simulink model "REL"  (R2022a)
settings: Solver=FixedStepDiscrete  StartTime=0.0  StopTime=10.0  FixedStep=0.01  RelTol=1e-3
libraries: simulink x4, DoorRatSts x4, DoorRlsDriver x4, DoorRlsReq x4
(part 2 of 2)

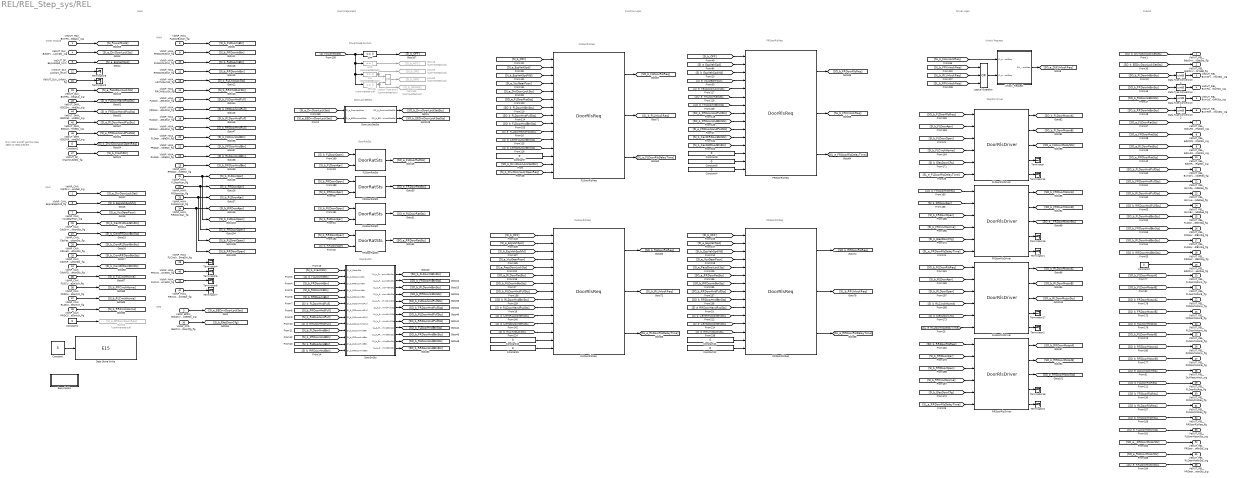
== system REL/REL_Step_sys/REL ==
  note: Only NFC and BT got this Req
      | //830 no need present
  note: CAN
  note: HWA
  note: Function Logic
  note: Input
  note: Output
  note: Input Preprocess
  note: Other Module
  note: CFG
  note: PowerMode Divition
  note: DoorLockSetSts
  note: DoorRatSts
  note: Driver Logic
  note: Unlock Request
  note: DoorRls Driver
  note: FLDoorRlsReq
  note: FRDoorRlsReq
  note: RLDoorRlsReq
  note: RRDoorRlsReq
  note: DoorSwSts
  VeOUT_PDU_BcmPowerStatusFeedback_sig : Inport
  VeINP_CAN_CdcDrvrDoorLockSet_sig : Inport  Port=2
  VeINP_EPRM_BdcDrvrDoorLockSetSts_sig : Inport  Port=3
  VeOUT_DLK_BdcDrvrDoorLockSts_sig : Inport  Port=4
  VeOUT_SP_EspVehSpd_kmh : Inport  Port=5
  VbINP_CAN_EspVehSpdVld_flg : Inport  Port=6
  VeINP_CAN_VcuGearPosn_sig : Inport  Port=7
  VbINP_HWA_FLDoorButton_flg : Inport  Port=8
  VbINP_HWA_FRDoorButton_flg : Inport  Port=9
  VbINP_HWA_RLDoorButton_flg : Inport  Port=10
  VbINP_HWA_RRDoorButton_flg : Inport  Port=11
  VmOUT_DLK_LockSrc_enum : Inport  Port=12
  VbINP_HWA_LRChildLckSt_flg : Inport  Port=13
  VbINP_HWA_RRChildLckSt_flg : Inport  Port=14
  VbOUT_DLK_Unlock_flg : Inport  Port=15
  VbINP_HWA_FLDoorOutButton_flg : Inport  Port=16
  VbINP_HWA_FRDoorOutButton_flg : Inport  Port=17
  VbINP_HWA_RLDoorOutButton_flg : Inport  Port=18
  VbINP_HWA_RRDoorOutButton_flg : Inport  Port=19
  VbINP_HWA_FLDoorHandleSW_flg : Inport  Port=20
  VbINP_HWA_FRDoorHandleSW_flg : Inport  Port=21
  VbINP_HWA_RLDoorHandleSW_flg : Inport  Port=22
  VbINP_HWA_RRDoorHandleSW_flg : Inport  Port=23
  VbINP_CAN_CdcAllDoorOpenButtonSts_flg : Inport  Port=24
  VeOUT_DLK_BCMPassengerDoorLockStatus_sig : Inport  Port=25
  VbINP_CAN_CdcDrvrDoorButtonSts_flg : Inport  Port=26
  VbINP_CAN_CdcPassDoorButtonSts_flg : Inport  Port=27
  VbINP_CAN_CdcLeReDoorButtonSts_flg : Inport  Port=28
  VbINP_CAN_CdcRiReDoorButtonSts_flg : Inport  Port=29
  VbINP_CFG_ElectricalDoorCfg_flg : Inport  Port=30
  VbINP_HWA_FLDoorAjar_flg : Inport  Port=31
  VbINP_HWA_FRDoorAjar_flg : Inport  Port=32
  VbINP_HWA_RLDoorAjar_flg : Inport  Port=33
  VbINP_HWA_RRDoorAjar_flg : Inport  Port=34
  VbINP_CAN_FLDCUCinchHomeSwitch_flg : Inport  Port=35
  VbINP_CAN_FRDCUCinchHomeSwitch_flg : Inport  Port=36
  VbINP_CAN_RLDCUCinchHomeSwitch_flg : Inport  Port=37
  VbINP_CAN_RRDCUCinchHomeSwitch_flg : Inport  Port=38
  VbINP_HWA_FLCinchHomeSW_flg : Inport  Port=39
  VbINP_HWA_FRCinchHomeSW_flg : Inport  Port=40
  VbINP_HWA_RLCinchHomeSW_flg : Inport  Port=41
  VbINP_HWA_RRCinchHomeSW_flg : Inport  Port=42
  VeOUT_DHM_BDCDrvrDoorHndSts_sig : Inport  Port=43
  VeOUT_DHM_BDCPassDoorHndSts_sig : Inport  Port=44
  VeOUT_DHM_BDCLeReDoorHndSts_sig : Inport  Port=45
  VeOUT_DHM_BDCRiReDoorHndSts_sig : Inport  Port=46
  VbOUT_SP_CrashOutpSts_flg : Inport  Port=47
  ACC : simulink/Logic and Bit Operations/Compare To Constant  Commented=on  relop===  const=1  OutDataTypeStr=boolean
  Constant : Constant  Value=5
  Constant1 : Constant  Value=0  OutDataTypeStr=uint8
  Constant{2..4,6..12} (10 alike) : Constant  Value=0  OutDataTypeStr=boolean
  Data Store Write : DataStoreWrite  DataStoreName=E15  IndexOptions=Index vector (dialog)  Indices=1  OutputSizes=1
  Data Type Conversion{,1..2,4} (4 alike) : DataTypeConversion  OutDataTypeStr=uint8  SaturateOnIntegerOverflow=off  RndMeth=Floor
  DoorLockSetSts : Stateflow chart  TreatAsAtomicUnit=on
  DoorSwSts : Stateflow chart  TreatAsAtomicUnit=on
  FLDoorRatSts : DoorRatSts/DoorRatSts  SystemSampleTime=-1  VariantActivationTime=update diagram  Latency=0  AutoFrameSizeCalculation=off
  FLDoorRlsDriver : DoorRlsDriver/DoorRlsDriver  SystemSampleTime=-1  VariantActivationTime=update diagram  Latency=0  AutoFrameSizeCalculation=off
  FLDoorRlsReq : DoorRlsReq/DoorRlsReq  SystemSampleTime=-1  VariantActivationTime=update diagram  Latency=0  AutoFrameSizeCalculation=off
  FRDoorRatSts : DoorRatSts/DoorRatSts  SystemSampleTime=-1  VariantActivationTime=update diagram  Latency=0  AutoFrameSizeCalculation=off
  FRDoorRlsDriver : DoorRlsDriver/DoorRlsDriver  SystemSampleTime=-1  VariantActivationTime=update diagram  Latency=0  AutoFrameSizeCalculation=off
  FRDoorRlsReq : DoorRlsReq/DoorRlsReq  SystemSampleTime=-1  VariantActivationTime=update diagram  Latency=0  AutoFrameSizeCalculation=off
  GRANK : simulink/Logic and Bit Operations/Compare To Constant  Commented=on  relop===  const=3  OutDataTypeStr=boolean
  Goto106 : Goto  Commented=on  GotoTag=SI_b_GRANK
  Goto48 : Goto  Commented=on  GotoTag=SI_b_ACC
  Goto56 : Goto  Commented=on  GotoTag=SI_e_BTDoorOpenReq
  Goto58 : Goto  Commented=on  GotoTag=SI_b_ON
  Goto69 : Goto  Commented=on  GotoTag=SI_b_IGN
  Logical Operator3 : Logic  Commented=on  Operator=OR  AllPortsSameDT=off  OutDataTypeStr=boolean
  Logical Operator : Logic  Operator=OR  Inputs=3  OutDataTypeStr=boolean
  "OFF " : simulink/Logic and Bit Operations/Compare To Constant  relop===  const=0  OutDataTypeStr=boolean
  ON : simulink/Logic and Bit Operations/Compare To Constant  Commented=on  relop===  const=2  OutDataTypeStr=boolean
  RLDoorRatSts : DoorRatSts/DoorRatSts  SystemSampleTime=-1  VariantActivationTime=update diagram  Latency=0  AutoFrameSizeCalculation=off
  RLDoorRlsDriver : DoorRlsDriver/DoorRlsDriver  SystemSampleTime=-1  VariantActivationTime=update diagram  Latency=0  AutoFrameSizeCalculation=off
  RLDoorRlsReq : DoorRlsReq/DoorRlsReq  SystemSampleTime=-1  VariantActivationTime=update diagram  Latency=0  AutoFrameSizeCalculation=off
  RRDoorRatSts : DoorRatSts/DoorRatSts  SystemSampleTime=-1  VariantActivationTime=update diagram  Latency=0  AutoFrameSizeCalculation=off
  RRDoorRlsDriver : DoorRlsDriver/DoorRlsDriver  SystemSampleTime=-1  VariantActivationTime=update diagram  Latency=0  AutoFrameSizeCalculation=off
  RRDoorRlsReq : DoorRlsReq/DoorRlsReq  SystemSampleTime=-1  VariantActivationTime=update diagram  Latency=0  AutoFrameSizeCalculation=off
  Recycle Bin : Subsystem
  Terminator{,1..9,15..18} (14 alike) : Terminator
  Unlock_Request : Stateflow chart  TreatAsAtomicUnit=on
  VbOUT_REL_BdcDrvrDoorLockSetSts_flg : Outport
  VbOUT_REL_BdcDrvrDoorLockSetStsToEE_flg : Outport  Port=2
  VeOUT_REL_BcmDrvrDoorSwtSts_sig : Outport  Port=3
  VeOUT_REL_BcmPassDoorSwtSts_sig : Outport  Port=4  OutDataTypeStr=uint8
  VeOUT_REL_BcmLeReDoorSwtSts_sig : Outport  Port=5  OutDataTypeStr=uint8
  VeOUT_REL_BcmRiReDoorSwtSts_sig : Outport  Port=6  OutDataTypeStr=uint8
  VeOUT_REL_BdcLFDoorRatSts_sig : Outport  Port=7
  VeOUT_REL_BdcRFDoorRatSts_sig : Outport  Port=8
  VeOUT_REL_BdcLRDoorRatSts_sig : Outport  Port=9
  VeOUT_REL_BdcRRDoorRatSts_sig : Outport  Port=10
  VbOUT_REL_BcmDrvrDoorHandleReq_flg : Outport  Port=11
  VbOUT_REL_BcmPassDoorHandleReq_flg : Outport  Port=12
  VbOUT_REL_BcmLeReDoorHandleReq_flg : Outport  Port=13
  VbOUT_REL_BcmBcmRiReDoorHandleReq_flg : Outport  Port=14
  VbOUT_REL_FLDoorHndlBtnSig_flg : Outport  Port=15
  VbOUT_REL_FRDoorHndlBtnSig_flg : Outport  Port=16
  VbOUT_REL_RLDoorHndlBtnSig_flg : Outport  Port=17
  VbOUT_REL_RRDoorHndlBtnSig_flg : Outport  Port=18
  VbOUT_REL_BdcDrvrDoorLockOpenReq_flg : Outport  Port=19
  VbOUT_REL_FLDoorMotorA_flg : Outport  Port=20
  VbOUT_REL_FLDoorMotorB_flg : Outport  Port=21
  VbOUT_REL_FRDoorMotorA_flg : Outport  Port=22
  VbOUT_REL_FRDoorMotorB_flg : Outport  Port=23
  VbOUT_REL_RLDoorMotorA_flg : Outport  Port=24
  VbOUT_REL_RLDoorMotorB_flg : Outport  Port=25
  VbOUT_REL_RRDoorMotorA_flg : Outport  Port=26
  VbOUT_REL_RRDoorMotorB_flg : Outport  Port=27
  VeOUT_REL_DLKReqUnlock_sig : Outport  Port=28
  VbOUT_REL_FLDoorRlsReq_flg : Outport  Port=29
  VbOUT_REL_FRDoorRlsReq_flg : Outport  Port=30
  VbOUT_REL_RLDoorRlsReq_flg : Outport  Port=31
  VbOUT_REL_RRDoorRlsReq_flg : Outport  Port=32
  VeOUT_REL_FLDoorMotorSts_sig : Outport  Port=33
  VeOUT_REL_FRDoorMotorSts_sig : Outport  Port=34
  VeOUT_REL_RLDoorMotorSts_sig : Outport  Port=35
  VeOUT_REL_RRDoorMotorSts_sig : Outport  Port=36
  wires:
  "OFF "/1 -> [SI_b_OFF]
  [SI_PowerMode] -> "OFF "/1, GRANK/1, ON/1, ACC/1
  ON/1 -> Goto58/1, Logical Operator3/1
  GRANK/1 -> Goto106/1, Logical Operator3/2
  Logical Operator3/1 -> Goto69/1
  ACC/1 -> Goto48/1
  VeINP_EPRM_BdcDrvrDoorLockSetSts_sig/1 -> [SI_e_EEDrvrDoorLockSet]
  [SO_b_DrvrDoorLockSetSts] -> VbOUT_REL_BdcDrvrDoorLockSetSts_flg/1
  DoorLockSetSts/1(SO_b_DoorLockSetSts) -> [SO_b_DrvrDoorLockSetSts]
  VeINP_CAN_CdcDrvrDoorLockSet_sig/1 -> [SI_e_DrvDoorLockSet]
  [SI_e_EEDrvrDoorLockSet] -> DoorLockSetSts/2(SI_e_EEDoorLockSet)
  VeOUT_DLK_BdcDrvrDoorLockSts_sig/1 -> [SI_e_DrvDoorLockSts]
  VeOUT_SP_EspVehSpd_kmh/1 -> [SI_e_EspVehSpd]
  VbINP_CAN_EspVehSpdVld_flg/1 -> [SI_b_EspVehSpdVld]
  VbINP_HWA_FLDoorButton_flg/1 -> [SI_b_FLDoorInBtn]
  VeINP_CAN_VcuGearPosn_sig/1 -> [SI_e_VcuGearPosn]
  VeOUT_DLK_BCMPassengerDoorLockStatus_sig/1 -> [SI_e_PassDoorLockSts]
  VbINP_HWA_FRDoorButton_flg/1 -> [SI_b_FRDoorInBtn]
  VbINP_HWA_LRChildLckSt_flg/1 -> [SI_b_RLChildLckSts]
  VbINP_HWA_RRChildLckSt_flg/1 -> [SI_b_RRChildLckSts]
  VbINP_CAN_CdcDrvrDoorButtonSts_flg/1 -> [SI_b_CentFLDoorBtnSts]
  VbINP_CAN_CdcPassDoorButtonSts_flg/1 -> [SI_b_CentFRDoorBtnSts]
  VbINP_CAN_CdcLeReDoorButtonSts_flg/1 -> [SI_b_CentRLDoorBtnSts]
  VbINP_CAN_CdcRiReDoorButtonSts_flg/1 -> [SI_b_CentRRDoorBtnSts]
  VbINP_HWA_RLDoorButton_flg/1 -> [SI_b_RLDoorInBtn]
  VbINP_HWA_RRDoorButton_flg/1 -> [SI_b_RRDoorInBtn]
  VbINP_HWA_FLDoorAjar_flg/1 -> [SI_b_FLDoorOpen], [SI_b_FLDoorAjar]
  VbINP_HWA_FRDoorAjar_flg/1 -> [SI_b_FRDoorOpen], [SI_b_FRDoorAjar]
  VbINP_HWA_RLDoorAjar_flg/1 -> [SI_b_RLDoorOpen], [SI_b_RLDoorAjar]
  VbINP_HWA_RRDoorAjar_flg/1 -> [SI_b_RRDoorOpen], [SI_b_RRDoorAjar]
  [SI_b_FLDoorOpen] -> FLDoorRatSts/1
  [SI_b_RRDoorAjar] -> RRDoorRatSts/2
  [SI_b_RLDoorAjar] -> RLDoorRatSts/2
  [SI_b_FRDoorAjar] -> FRDoorRatSts/2
  [SI_b_FLDoorAjar] -> FLDoorRatSts/2
  [SI_b_FRDoorOpen] -> FRDoorRatSts/1
  [SI_b_RLDoorOpen] -> RLDoorRatSts/1
  [SI_b_RRDoorOpen] -> RRDoorRatSts/1
  [SO_e_FLDoorRatSts] -> VeOUT_REL_BdcLFDoorRatSts_sig/1
  [SO_e_FRDoorRatSts] -> VeOUT_REL_BdcRFDoorRatSts_sig/1
  [SO_e_RLDoorRatSts] -> VeOUT_REL_BdcLRDoorRatSts_sig/1
  [SO_e_RRDoorRatSts] -> VeOUT_REL_BdcRRDoorRatSts_sig/1
  FLDoorRatSts/1 -> [SO_e_FLDoorRatSts]
  FRDoorRatSts/1 -> [SO_e_FRDoorRatSts]
  RRDoorRatSts/1 -> [SO_e_RRDoorRatSts]
  RLDoorRatSts/1 -> [SO_e_RLDoorRatSts]
  [SO_b_FRDoorInBtnSts] -> Data Type Conversion/1
  [SO_b_RLDoorInBtnSts] -> Data Type Conversion1/1
  [SO_b_RRDoorInBtnSts] -> Data Type Conversion2/1
  [SO_e_DLKUnlockReq] -> VeOUT_REL_DLKReqUnlock_sig/1
  VbINP_HWA_FLDoorHandleSW_flg/1 -> [SI_b_FLDoorHndBtn]
  VbINP_HWA_FRDoorHandleSW_flg/1 -> [SI_b_FRDoorHndBtn]
  VbINP_HWA_RLDoorHandleSW_flg/1 -> [SI_b_RLDoorHndBtn]
  VbINP_HWA_RRDoorHandleSW_flg/1 -> [SI_b_RRDoorHndBtn]
  [SO_b_FLDoorHndPullSts] -> VbOUT_REL_BcmDrvrDoorHandleReq_flg/1
  [SO_b_FRDoorHndPullSts] -> VbOUT_REL_BcmPassDoorHandleReq_flg/1
  [SO_b_RLDoorHndPullSts] -> VbOUT_REL_BcmLeReDoorHandleReq_flg/1
  [SO_b_RRDoorHndPullSts] -> VbOUT_REL_BcmBcmRiReDoorHandleReq_flg/1
  VbINP_HWA_FLDoorOutButton_flg/1 -> [SI_b_FLDoorHndPull]
  VbINP_HWA_FRDoorOutButton_flg/1 -> [SI_b_FRDoorHndPull]
  VbINP_HWA_RLDoorOutButton_flg/1 -> [SI_b_RLDoorHndPull]
  VbINP_HWA_RRDoorOutButton_flg/1 -> [SI_b_RRDoorHndPull]
  [SO_b_FLDoorHndBtnSts] -> VbOUT_REL_FLDoorHndlBtnSig_flg/1
  [SO_b_FRDoorHndBtnSts] -> VbOUT_REL_FRDoorHndlBtnSig_flg/1
  [SO_b_RLDoorHndBtnSts] -> VbOUT_REL_RLDoorHndlBtnSig_flg/1
  [SO_b_RRDoorHndBtnSts] -> VbOUT_REL_RRDoorHndlBtnSig_flg/1
  VeOUT_PDU_BcmPowerStatusFeedback_sig/1 -> [SI_PowerMode]
  Constant2/1 -> [SI_b_DrvrDoorLockOpenReq]
  VeOUT_DHM_BDCDrvrDoorHndSts_sig/1 -> [SI_e_FLDoorHandPosSts]
  Constant1/1 -> Goto56/1
  VbINP_CAN_CdcAllDoorOpenButtonSts_flg/1 -> [SI_b_CentAllDoorBtnSts]
  VeOUT_DHM_BDCPassDoorHndSts_sig/1 -> [SI_e_FRDoorHandPosSts]
  VeOUT_DHM_BDCLeReDoorHndSts_sig/1 -> [SI_e_RLDoorHandPosSts]
  VeOUT_DHM_BDCRiReDoorHndSts_sig/1 -> [SI_e_RRDoorHandPosSts]
  Constant3/1 -> VbOUT_REL_BdcDrvrDoorLockOpenReq_flg/1
  [SO_b_FLDoorMotorA] -> VbOUT_REL_FLDoorMotorA_flg/1
  [SO_b_FLDoorMotorB] -> VbOUT_REL_FLDoorMotorB_flg/1
  FLDoorRlsDriver/2 -> [SO_b_FLDoorMotorB]
  FLDoorRlsDriver/1 -> [SO_b_FLDoorMotorA]
  [SO_b_FLDoorRlsReq] -> VbOUT_REL_FLDoorRlsReq_flg/1
  [SO_b_FRDoorRlsReq] -> VbOUT_REL_FRDoorRlsReq_flg/1
  [SO_b_RLDoorRlsReq] -> VbOUT_REL_RLDoorRlsReq_flg/1
  [SO_b_RRDoorRlsReq] -> VbOUT_REL_RRDoorRlsReq_flg/1
  [SO_b_FLDoorRlsReq] -> FLDoorRlsDriver/1
  [SI_b_FLDoorAjar] -> FLDoorRlsDriver/2
  VbINP_CAN_FLDCUCinchHomeSwitch_flg/1 -> [SI_b_FLCinchHome]
  VbINP_CAN_FRDCUCinchHomeSwitch_flg/1 -> [SI_b_FRCinchHome]
  VbINP_CAN_RLDCUCinchHomeSwitch_flg/1 -> [SI_b_RLCinchHome]
  VbINP_CAN_RRDCUCinchHomeSwitch_flg/1 -> [SI_b_RRCinchHome]
  [SO_b_FRDoorRlsReq] -> FRDoorRlsDriver/1
  [SI_b_FLCinchHome] -> FLDoorRlsDriver/4
  VbINP_CFG_ElectricalDoorCfg_flg/1 -> [SI_b_ElecDoorCfg]
  [SI_b_ElecDoorCfg] -> FLDoorRlsDriver/5
  [SO_b_FRDoorMotorB] -> VbOUT_REL_FRDoorMotorB_flg/1
  [SO_b_RLDoorMotorB] -> VbOUT_REL_RLDoorMotorB_flg/1
  [SO_b_RRDoorMotorB] -> VbOUT_REL_RRDoorMotorB_flg/1
  [SO_b_FRDoorMotorA] -> VbOUT_REL_FRDoorMotorA_flg/1
  [SO_b_RLDoorMotorA] -> VbOUT_REL_RLDoorMotorA_flg/1
  [SO_b_RRDoorMotorA] -> VbOUT_REL_RRDoorMotorA_flg/1
  [SO_e_FLDoorMotorSts] -> VeOUT_REL_FLDoorMotorSts_sig/1
  [SO_e__FRDoorMotorSts] -> VeOUT_REL_FRDoorMotorSts_sig/1
  [SO_e_RLDoorMotorSts] -> VeOUT_REL_RLDoorMotorSts_sig/1
  [SO_e_RRDoorMotorSts] -> VeOUT_REL_RRDoorMotorSts_sig/1
  FLDoorRlsDriver/3 -> [SO_e_FLDoorMotorSts]
  FLDoorRlsDriver/4 -> Terminator/1
  FRDoorRlsDriver/5 -> Terminator1/1
  RLDoorRlsDriver/5 -> Terminator2/1
  RRDoorRlsDriver/5 -> Terminator3/1
  VbINP_HWA_FLCinchHomeSW_flg/1 -> Terminator4/1
  VbINP_HWA_FRCinchHomeSW_flg/1 -> Terminator5/1
  VbINP_HWA_RLCinchHomeSW_flg/1 -> Terminator6/1
  VbINP_HWA_RRCinchHomeSW_flg/1 -> Terminator7/1
  VmOUT_DLK_LockSrc_enum/1 -> Terminator8/1
  VbOUT_DLK_Unlock_flg/1 -> Terminator9/1
  VbOUT_SP_CrashOutpSts_flg/1 -> [SI_b_CrashSts]
  [SI_b_FLDoorOpen] -> FLDoorRlsDriver/3
  [SO_b_EEDrvDoorLockSetSts] -> VbOUT_REL_BdcDrvrDoorLockSetStsToEE_flg/1
  DoorLockSetSts/2(SO_b_EEDoorLockSetSts) -> [SO_b_EEDrvDoorLockSetSts]
  Data Type Conversion/1 -> VeOUT_REL_BcmPassDoorSwtSts_sig/1
  Data Type Conversion1/1 -> VeOUT_REL_BcmLeReDoorSwtSts_sig/1
  Data Type Conversion2/1 -> VeOUT_REL_BcmRiReDoorSwtSts_sig/1
  [SO_b_FLDoorInBtnSts] -> Data Type Conversion4/1
  Data Type Conversion4/1 -> VeOUT_REL_BcmDrvrDoorSwtSts_sig/1
  Unlock_Request/1(SO_e_UnlockReq) -> [SO_e_DLKUnlockReq]
  FLDoorRlsReq/1 -> [SO_b_FLDoorRlsReq]
  FLDoorRlsReq/2 -> [SL_b_FLUnlockReq]
  FRDoorRlsReq/1 -> [SO_b_FRDoorRlsReq]
  FRDoorRlsReq/2 -> [SL_b_FRUnlockReq]
  RLDoorRlsReq/1 -> [SO_b_RLDoorRlsReq]
  RLDoorRlsReq/2 -> [SL_b_RLUnlockReq]
  RRDoorRlsReq/1 -> [SO_b_RRDoorRlsReq]
  RRDoorRlsReq/2 -> [SL_b_RRUnlockReq]
  [SL_b_FLUnlockReq] -> Unlock_Request/1(SI_b_DrvUnlockReq)
  [SL_b_FRUnlockReq] -> Logical Operator/1
  [SL_b_RLUnlockReq] -> Logical Operator/2
  [SL_b_RRUnlockReq] -> Logical Operator/3
  Logical Operator/1 -> Unlock_Request/2(SI_b_PassUnlockReq)
  [SI_e_DrvDoorLockSet] -> DoorLockSetSts/1(SI_e_DoorLockSet)
  FLDoorRlsDriver/5 -> Terminator15/1
  [SI_b_FRDoorOpen] -> FRDoorRlsDriver/3
  [SI_b_FRCinchHome] -> FRDoorRlsDriver/4
  [SI_b_ElecDoorCfg] -> FRDoorRlsDriver/5
  [SI_b_FRDoorAjar] -> FRDoorRlsDriver/2
  FRDoorRlsDriver/2 -> [SO_b_FRDoorMotorB]
  FRDoorRlsDriver/1 -> [SO_b_FRDoorMotorA]
  FRDoorRlsDriver/3 -> [SO_e__FRDoorMotorSts]
  FRDoorRlsDriver/4 -> Terminator16/1
  [SO_b_RLDoorRlsReq] -> RLDoorRlsDriver/1
  [SI_b_RLDoorAjar] -> RLDoorRlsDriver/2
  [SI_b_RLDoorOpen] -> RLDoorRlsDriver/3
  [SI_b_RLCinchHome] -> RLDoorRlsDriver/4
  [SI_b_ElecDoorCfg] -> RLDoorRlsDriver/5
  RLDoorRlsDriver/1 -> [SO_b_RLDoorMotorA]
  RLDoorRlsDriver/3 -> [SO_e_RLDoorMotorSts]
  RLDoorRlsDriver/2 -> [SO_b_RLDoorMotorB]
  RLDoorRlsDriver/4 -> Terminator17/1
  [SO_b_RRDoorRlsReq] -> RRDoorRlsDriver/1
  [SI_b_RRDoorAjar] -> RRDoorRlsDriver/2
  [SI_b_RRDoorOpen] -> RRDoorRlsDriver/3
  [SI_b_RRCinchHome] -> RRDoorRlsDriver/4
  [SI_b_ElecDoorCfg] -> RRDoorRlsDriver/5
  RRDoorRlsDriver/2 -> [SO_b_RRDoorMotorB]
  RRDoorRlsDriver/1 -> [SO_b_RRDoorMotorA]
  RRDoorRlsDriver/3 -> [SO_e_RRDoorMotorSts]
  RRDoorRlsDriver/4 -> Terminator18/1
  [SO_b_FLDoorHndPullSts] -> FLDoorRlsReq/8
  [SO_b_FLDoorHndBtnSts] -> FLDoorRlsReq/9
  [SI_b_OFF] -> FLDoorRlsReq/1
  [SI_e_EspVehSpd] -> FLDoorRlsReq/2
  [SI_b_EspVehSpdVld] -> FLDoorRlsReq/3
  [SI_e_VcuGearPosn] -> FLDoorRlsReq/4
  [SI_e_DrvDoorLockSts] -> FLDoorRlsReq/5
  [SO_e_FLDoorRatSts] -> FLDoorRlsReq/6
  [SO_b_FLDoorInBtnSts] -> FLDoorRlsReq/7
  [SO_b_RLDoorHndPullSts] -> RLDoorRlsReq/8
  [SI_b_OFF] -> RLDoorRlsReq/1
  [SI_e_EspVehSpd] -> RLDoorRlsReq/2
  [SI_b_EspVehSpdVld] -> RLDoorRlsReq/3
  [SI_e_VcuGearPosn] -> RLDoorRlsReq/4
  [SO_b_RLDoorHndBtnSts] -> RLDoorRlsReq/9
  [SI_e_PassDoorLockSts] -> RLDoorRlsReq/5
  [SO_e_RLDoorRatSts] -> RLDoorRlsReq/6
  [SO_b_RLDoorInBtnSts] -> RLDoorRlsReq/7
  [SI_b_OFF] -> FRDoorRlsReq/1
  [SI_e_EspVehSpd] -> FRDoorRlsReq/2
  [SI_b_EspVehSpdVld] -> FRDoorRlsReq/3
  [SI_e_VcuGearPosn] -> FRDoorRlsReq/4
  [SO_b_FRDoorHndPullSts] -> FRDoorRlsReq/8
  [SO_b_FRDoorHndBtnSts] -> FRDoorRlsReq/9
  [SI_e_PassDoorLockSts] -> FRDoorRlsReq/5
  [SO_e_FRDoorRatSts] -> FRDoorRlsReq/6
  [SO_b_FRDoorInBtnSts] -> FRDoorRlsReq/7
  [SI_b_OFF] -> RRDoorRlsReq/1
  [SI_e_EspVehSpd] -> RRDoorRlsReq/2
  [SI_b_EspVehSpdVld] -> RRDoorRlsReq/3
  [SI_e_VcuGearPosn] -> RRDoorRlsReq/4
  [SI_e_PassDoorLockSts] -> RRDoorRlsReq/5
  [SO_e_RRDoorRatSts] -> RRDoorRlsReq/6
  [SO_b_RRDoorInBtnSts] -> RRDoorRlsReq/7
  [SO_b_RRDoorHndPullSts] -> RRDoorRlsReq/8
  [SO_b_RRDoorHndBtnSts] -> RRDoorRlsReq/9
  DoorSwSts/1(SL_b_FLDoorInBtnSts) -> [SO_b_FLDoorInBtnSts]
  [SI_b_FRDoorInBtn] -> DoorSwSts/3(SI_b_FRDoorInBtn)
  [SI_b_FLDoorInBtn] -> DoorSwSts/2(SI_b_FLDoorInBtn)
  [SI_b_CrashSts] -> DoorSwSts/1(SI_b_CrashSts)
  [SI_b_RLDoorInBtn] -> DoorSwSts/4(SI_b_RLDoorInBtn)
  [SI_b_RRDoorInBtn] -> DoorSwSts/5(SI_b_RRDoorInBtn)
  [SI_b_FLDoorHndPull] -> DoorSwSts/6(SI_b_FLDoorHndPull)
  [SI_b_FRDoorHndPull] -> DoorSwSts/7(SI_b_FRDoorHndPull)
  [SI_b_RLDoorHndPull] -> DoorSwSts/8(SI_b_RLDoorHndPull)
  [SI_b_RRDoorHndPull] -> DoorSwSts/9(SI_b_RRDoorHndPull)
  [SI_b_FLDoorHndBtn] -> DoorSwSts/10(SI_b_FLDoorHndBtn)
  [SI_b_FRDoorHndBtn] -> DoorSwSts/11(SI_b_FRDoorHndBtn)
  [SI_b_RLDoorHndBtn] -> DoorSwSts/12(SI_b_RLDoorHndBtn)
  [SI_b_RRDoorHndBtn] -> DoorSwSts/13(SI_b_RRDoorHndBtn)
  DoorSwSts/2(SL_b_FRDoorInBtnSts) -> [SO_b_FRDoorInBtnSts]
  DoorSwSts/3(SL_b_RLDoorInBtnSts) -> [SO_b_RLDoorInBtnSts]
  DoorSwSts/4(SL_b_RRDoorInBtnSts) -> [SO_b_RRDoorInBtnSts]
  DoorSwSts/5(SL_b_FLDoorHndPullSts) -> [SO_b_FLDoorHndPullSts]
  DoorSwSts/6(SL_b_FRDoorHndPullSts) -> [SO_b_FRDoorHndPullSts]
  DoorSwSts/7(SL_b_RLDoorHndPullSts) -> [SO_b_RLDoorHndPullSts]
  DoorSwSts/8(SL_b_RRDoorHndPullSts) -> [SO_b_RRDoorHndPullSts]
  DoorSwSts/9(SL_b_FLDoorHndBtnSts) -> [SO_b_FLDoorHndBtnSts]
  DoorSwSts/10(SL_b_FRDoorHndBtnSts) -> [SO_b_FRDoorHndBtnSts]
  DoorSwSts/11(SL_b_RLDoorHndBtnSts) -> [SO_b_RLDoorHndBtnSts]
  DoorSwSts/12(SL_b_RRDoorHndBtnSts) -> [SO_b_RRDoorHndBtnSts]
  [SO_b_DrvrDoorLockSetSts] -> FLDoorRlsReq/14
  [SI_b_CentFLDoorBtnSts] -> FLDoorRlsReq/11
  [SI_b_CentAllDoorBtnSts] -> FLDoorRlsReq/12
  Constant7/1 -> FLDoorRlsReq/13
  [SI_e_FLDoorHandPosSts] -> FLDoorRlsReq/10
  Constant8/1 -> FRDoorRlsReq/13
  Constant9/1 -> FRDoorRlsReq/14
  [SI_b_CentFRDoorBtnSts] -> FRDoorRlsReq/11
  [SI_b_CentAllDoorBtnSts] -> FRDoorRlsReq/12
  [SI_e_FRDoorHandPosSts] -> FRDoorRlsReq/10
  [SI_b_CentAllDoorBtnSts] -> RLDoorRlsReq/12
  [SI_e_RLDoorHandPosSts] -> RLDoorRlsReq/10
  [SI_b_CentRLDoorBtnSts] -> RLDoorRlsReq/11
  [SI_b_RLChildLckSts] -> RLDoorRlsReq/13
  Constant10/1 -> RLDoorRlsReq/14
  [SI_b_CentAllDoorBtnSts] -> RRDoorRlsReq/12
  [SI_b_RRChildLckSts] -> RRDoorRlsReq/13
  Constant11/1 -> RRDoorRlsReq/14
  [SI_b_CentRRDoorBtnSts] -> RRDoorRlsReq/11
  [SI_e_RRDoorHandPosSts] -> RRDoorRlsReq/10
  FLDoorRlsReq/3 -> [SL_e_FLDoorRlsDelayTime]
  FRDoorRlsReq/3 -> [SL_e_FRDoorRlsDelayTime]
  RLDoorRlsReq/3 -> [SL_e_RLDoorRlsDelayTime]
  RRDoorRlsReq/3 -> [SL_e_RRDoorRlsDelayTime]
  [SL_e_FLDoorRlsDelayTime] -> FLDoorRlsDriver/6
  [SL_e_RLDoorRlsDelayTime] -> RLDoorRlsDriver/6
  [SL_e_FRDoorRlsDelayTime] -> FRDoorRlsDriver/6
  [SL_e_RRDoorRlsDelayTime] -> RRDoorRlsDriver/6
  [SI_b_DrvrDoorLockOpenReq] -> FLDoorRlsReq/15
  Constant4/1 -> FRDoorRlsReq/15
  Constant6/1 -> RLDoorRlsReq/15
  Constant12/1 -> RRDoorRlsReq/15
  Constant/1 -> Data Store Write/1

== system REL/REL_Step_sys/REL/Recycle Bin ==

== stateflow chart REL/REL_Step_sys/REL/DoorLockSetSts ==
  state DoorLockSet
    (default) -> (junction 127) : /* DoorLockSet */
        | {SL_e_DoorLockSetBackup = 0;}
    DoorLockSet -> (junction 127)
    (junction 127) -> (junction 128) [order 1] : [SI_e_DoorLockSet == 1 || ...
        | (SI_e_DoorLockSet == 0 && SL_e_DoorLockSetBackup == 1)]
    (junction 127) -> (junction 129) [order 2]
    (junction 128) -> (junction 136) : {SO_b_DoorLockSetSts = 1; ...
        | SO_b_EEDoorLockSetSts = 1; ...
        | SL_e_DoorLockSetBackup = 1}
    (junction 129) -> (junction 130) [order 1] : [SI_e_DoorLockSet == 2 || ...
        | (SI_e_DoorLockSet == 0 && SL_e_DoorLockSetBackup == 2)]
    (junction 129) -> (junction 131) [order 2]
    (junction 130) -> (junction 135) : {SO_b_DoorLockSetSts = 0; ...
        | SO_b_EEDoorLockSetSts = 0; ...
        | SL_e_DoorLockSetBackup = 2}
    (junction 131) -> (junction 132) [order 1] : [SI_e_EEDoorLockSet == 1]
    (junction 131) -> (junction 151) [order 2]
    (junction 132) -> (junction 134) : {SO_b_DoorLockSetSts = 1; ...
        | SO_b_EEDoorLockSetSts = 1;}
    (junction 151) -> (junction 159) [order 1] : [SI_e_EEDoorLockSet == 0]
    (junction 151) -> (junction 133) [order 2]
    (junction 159) -> (junction 160) : {SO_b_DoorLockSetSts = 0; ...
        | SO_b_EEDoorLockSetSts = 0;}
    (junction 160) -> (junction 133)
    (junction 134) -> (junction 160)
    (junction 135) -> (junction 134)
    (junction 136) -> (junction 135)
    (junction 133) -> (junction 137)
  data: SO_b_DoorLockSetSts output boolean; SI_e_DoorLockSet input uint8; SI_e_EEDoorLockSet input uint8; SO_b_EEDoorLockSetSts output boolean; SL_e_DoorLockSetBackup local uint8

== stateflow chart REL/REL_Step_sys/REL/Unlock_Request ==
  state REQ_SENT
    REQ_SENT -> (junction 56) [order 1]
    (junction 56) -> (junction 58) [order 1] : [SI_b_DrvUnlockReq == 1 &&...
        | SI_b_PassUnlockReq == 1]
    (junction 56) -> (junction 60) [order 2]
    (junction 58) -> (junction 91) : {SO_e_UnlockReq = 3;}
    (junction 60) -> (junction 62) [order 1] : [SI_b_DrvUnlockReq == 1&&...
        | SI_b_PassUnlockReq != 1]
    (junction 60) -> (junction 84) [order 2]
    (junction 62) -> (junction 93) : {SO_e_UnlockReq = 1;}
    (junction 84) -> (junction 83) [order 1] : [SI_b_DrvUnlockReq != 1 &&...
        | SI_b_PassUnlockReq == 1]
    (junction 84) -> (junction 88) [order 2] : {SO_e_UnlockReq = 0;}
    (junction 83) -> (junction 95) : {SO_e_UnlockReq = 2;}
  state Initial
    en:
    SO_e_UnlockReq = 0;
  (default) -> Initial
  Initial -> REQ_SENT : [hasChangedTo(SI_b_DrvUnlockReq, 1) ||...
      | hasChangedTo(SI_b_PassUnlockReq, 1)]
  REQ_SENT -> Initial [order 1] : [SI_b_DrvUnlockReq == 0 &&...
      | SI_b_PassUnlockReq == 0]
  data: SO_e_UnlockReq output uint8; SI_b_DrvUnlockReq input boolean; SI_b_PassUnlockReq input boolean

== stateflow chart REL/REL_Step_sys/REL/DoorSwSts ==
  state NoCrash
    en,du:
    SL_b_FLDoorInBtnSts = SI_b_FLDoorInBtn;
    SL_b_FRDoorInBtnSts = SI_b_FRDoorInBtn;
    SL_b_RLDoorInBtnSts = SI_b_RLDoorInBtn;
    SL_b_RRDoorInBtnSts = SI_b_RRDoorInBtn;
    SL_b_FLDoorHndPullSts = SI_b_FLDoorHndPull;
    SL_b_FRDoorHndPullSts = SI_b_FRDoorHndPull;
    SL_b_RLDoorHndPullSts = SI_b_RLDoorHndPull;
    SL_b_RRDoorHndPullSts = SI_b_RRDoorHndPull;
    SL_b_FLDoorHndBtnSts = SI_b_FLDoorHndBtn;
    SL_b_FRDoorHndBtnSts = SI_b_FRDoorHndBtn;
    SL_b_RLDoorHndBtnSts = SI_b_RLDoorHndBtn;
    SL_b_RRDoorHndBtnSts = SI_b_RRDoorHndBtn;
  state Crash
    en,du:
    SL_b_FLDoorInBtnSts = 0;
    SL_b_FRDoorInBtnSts = 0;
    SL_b_RLDoorInBtnSts = 0;
    SL_b_RRDoorInBtnSts = 0;
    SL_b_FLDoorHndPullSts = 0;
    SL_b_FRDoorHndPullSts = 0;
    SL_b_RLDoorHndPullSts = 0;
    SL_b_RRDoorHndPullSts = 0;
    SL_b_FLDoorHndBtnSts = 0;
    SL_b_FRDoorHndBtnSts = 0;
    SL_b_RLDoorHndBtnSts = 0;
    SL_b_RRDoorHndBtnSts = 0;
  (default) -> NoCrash
  NoCrash -> Crash : [hasChangedTo(SI_b_CrashSts, 1)]
  Crash -> NoCrash : [after(1000, tick)]
  data: SL_b_FLDoorInBtnSts output boolean; SI_b_CrashSts input boolean; SI_b_FLDoorInBtn input boolean; SI_b_FRDoorInBtn input boolean; SI_b_RLDoorInBtn input boolean; SI_b_RRDoorInBtn input boolean; SL_b_FRDoorInBtnSts output boolean; SL_b_RLDoorInBtnSts output boolean; SL_b_RRDoorInBtnSts output boolean; SI_b_FLDoorHndPull input boolean; SI_b_FRDoorHndPull input boolean; SI_b_RLDoorHndPull input boolean; SI_b_RRDoorHndPull input boolean; SI_b_FLDoorHndBtn input boolean; SI_b_FRDoorHndBtn input boolean; SI_b_RLDoorHndBtn input boolean; SI_b_RRDoorHndBtn input boolean; SL_b_FLDoorHndPullSts output boolean; SL_b_FRDoorHndPullSts output boolean; SL_b_RLDoorHndPullSts output boolean; SL_b_RRDoorHndPullSts output boolean; SL_b_FLDoorHndBtnSts output boolean; SL_b_FRDoorHndBtnSts output boolean; SL_b_RLDoorHndBtnSts output boolean; SL_b_RRDoorHndBtnSts output boolean
